simulink model "team8_simulink_model"  (R2019b)
settings: Solver=VariableStepAuto  StartTime=0.0  StopTime=10.0  RelTol=1e-3
libraries: fuzblock x1
settings Model: Creator=sewoods  LastModifiedBy=Jakub
settings SFSimCC: CustomCodeUndefinedFunction=UseInterfaceOnly

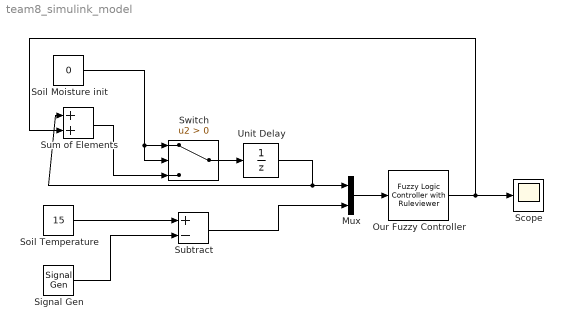
== system team8_simulink_model ==
  Mux : Mux  Inputs=2
  "Our Fuzzy Controller " : fuzblock/Fuzzy Logic  Controller  with Ruleviewer  fismatrix=team8_fuzzy_logic  Ts=0.1
  Scope : Scope
  "Signal Gen " : SignalGenerator  Amplitude=15  Frequency=0.5  Units=rad/sec
  "Soil Moisture init " : Constant  Value=0
  "Soil Temperature " : Constant  Value=15
  Subtract : Sum  Inputs=+-
  Sum of Elements : Sum
  Switch : Switch  Criteria=u2 > Threshold
  Unit Delay : UnitDelay  SampleTime=-1  HasFrameUpgradeWarning=on
  wires:
  "Soil Moisture init "/1 -> Switch/2, Switch/1
  Mux/1 -> "Our Fuzzy Controller "/1
  "Soil Temperature "/1 -> Subtract/1
  "Signal Gen "/1 -> Subtract/2
  Subtract/1 -> Mux/2
  "Our Fuzzy Controller "/1 -> Scope/1, Sum of Elements/2
  Switch/1 -> Unit Delay/1
  Unit Delay/1 -> Mux/1, Sum of Elements/1
  Sum of Elements/1 -> Switch/3
